simulink model "5-Behavior_State_Machine"  (R2021a)
settings: Solver=VariableStepAuto  StartTime=0.0  StopTime=10.0  RelTol=1e-3
settings Model: Creator=ibirl  LastModifiedBy=zht

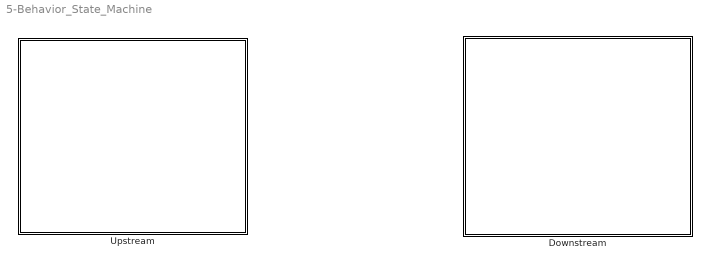
== system 5-Behavior_State_Machine ==
  Downstream : Stateflow chart  TreatAsAtomicUnit=on
  Upstream : Stateflow chart  TreatAsAtomicUnit=on

== stateflow chart 5-Behavior_State_Machine/Downstream ==
  state E
  state D
  state A
  state B
  state C
  E -> B [order 3] : (1)[0.9]{0}
  E -> A [order 2] : (1)[0.1*(1-pb)]{-1}
  E -> D [order 1] : (1)[0.1*pb]{-1}
  D -> E [order 1] : (A1)[1-pbd]{0}
  D -> D [order 2] : (1)[pbd]{0}
  C -> D [order 3] : (1)[pb]{-1}
  B -> D [order 4] : (1)[(0.6664)*pb]{-1}
  A -> D [order 3] : (0)[0.1*pb]{-1}
  C -> A [order 2] : (1)[1-pb]{-1}
  B -> A [order 3] : (1)[0.6664*(1-pb)]{-1}
  A -> B [order 2] : (0)[0.9]{0}
  B -> C [order 2] : (1)[0.2679]{0}
  A -> A [order 1] : (1)[0.1*(1-pb)]{-1}
  B -> B [order 1] : (1)[0.0657]{0}
  C -> C [order 1] : (1)[0]{0}

== stateflow chart 5-Behavior_State_Machine/Upstream ==
  state E
  state D
  state A
  state B
  state C
  E -> B [order 3] : (1)[0.9]{0}
  E -> A [order 2] : (1)[0.1*(1-ps)]{1}
  E -> D [order 1] : (1)[0.1*ps]{1}
  D -> E [order 1] : (A1)[1-psu]{0}
  C -> D [order 3] : (1)[ps]{1}
  D -> D [order 2] : (1)[psu]{0}
  B -> D [order 4] : (1)[(0.6664)*ps]{1}
  A -> D [order 3] : (0)[0.1*ps]{1}
  C -> A [order 2] : (1)[1-ps]{1}
  B -> A [order 3] : (1)[0.6664*(1-ps)]{1}
  A -> B [order 2] : (0)[0.9]{0}
  B -> C [order 2] : (1)[0.2679]{0}
  A -> A [order 1] : (1)[0.1*(1-ps)]{1}
  B -> B [order 1] : (1)[0.0657]{0}
  C -> C [order 1] : (1)[0]{0}
